simulink model "PWM_using_RSB"  (R2024a)
settings: Solver=VariableStepAuto  StartTime=0.0  StopTime=10.0  MaxStep=1e-4  RelTol=1e-3
libraries: simulink x1
settings Model: Creator=admin  LastModifiedBy=admin

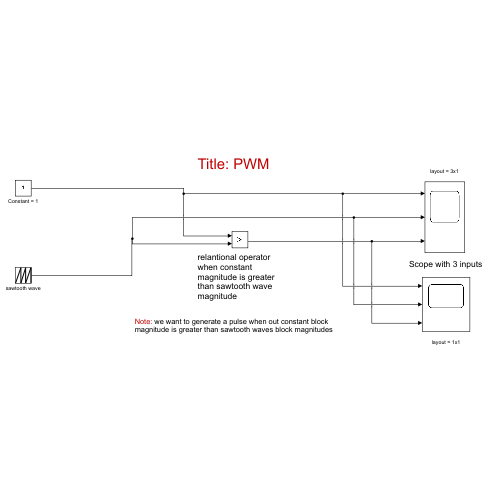
[thumbnail: Simulink's stored preview of the top-level diagram]
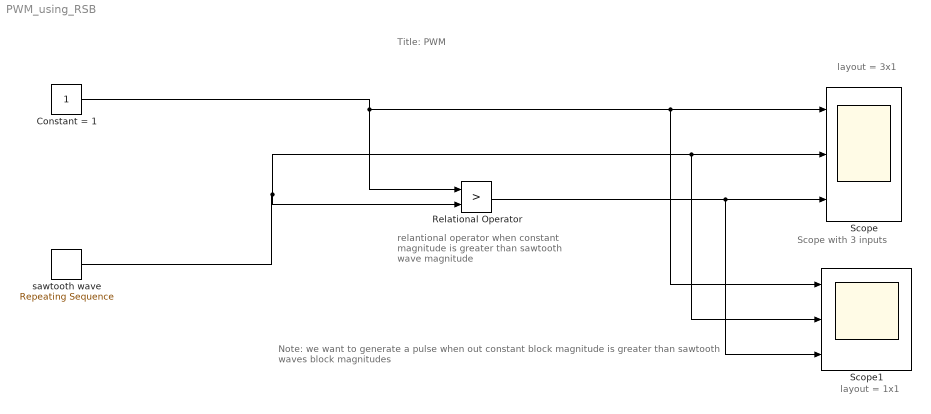
== system PWM_using_RSB ==
  note: layout = 3x1
  note: Title: PWM
  note: Note: we want to generate a pulse when out constant block magnitude is greater than sawtooth waves block magnitudes
  note: Scope with 3 inputs
  note: relantional operator
      | when constant magnitude is greater than sawtooth wave magnitude
  note: layout = 1x1
  Constant = 1 : Constant
  Relational Operator : RelationalOperator  Operator=>  OutDataTypeStr=boolean  RndMeth=Simplest  InputSameDT=off
  Scope : Scope  NumInputPorts=3
  Scope1 : Scope  NumInputPorts=3
  sawtooth wave : simulink/Sources/Repeating Sequence  rep_seq_t=[0 1]  rep_seq_y=[0 2]
  wires:
  Constant = 1/1 -> Relational Operator/1, Scope1/1, Scope/1
  sawtooth wave/1 -> Relational Operator/2, Scope1/2, Scope/2
  Relational Operator/1 -> Scope1/3, Scope/3
